simulink model "rev1BB"  (R2021a)
settings: Solver=FixedStepAuto  StartTime=0.0  StopTime=((((preLen+100+dataLenSymbols)*1+pad_first*3)*basePer))*2.5  RelTol=1e-3
values from neighbouring files (symbols this model uses):
  agcDesired = 0    [rev1BB_setup.m]
  agcStep = 2^-8    (= 0.00390625)    [rev1BB_setup.m]
  awgnSeed = abs(dBSnrRange(dBSnrInd)*1000+trial+10000000)    [plotBer.m]    (also in plotBerParSim.m; rev1BB_startup.m = 67)
  basePer = 1/baseFreq    (= 5e-08)    [rev1BB_setup.m]
  bitsPerSymbolHeader = log2(radixHeader)    [rev1BB_setup.m]
  bitsPerSymbolMax = log2(radixMax)    [rev1BB_setup.m]
  cefEarlyWarning = 256    [rev1BB_setup.m]
  cefLen = length(x_CEF)    [rev1BB_setup.m]
  cfoNcoWordLen = 16    [rev1BB_setup.m]
  channelFIR = zeros(1, round(maxSampleDelay)+1)    [rev1BB_simParams_setup.m]
  corr_peak_exclude_trigger = 1+corr_peak_trigger    (= 1.4)    [rev1BB_setup.m]
  corr_peak_trigger = 0.40    (= 0.4)    [rev1BB_setup.m]
  cr_i = 0.020    (= 0.02)    [rev1BB_setup.m]
  cr_i_preamp = 2^-9    (= 0.001953125)    [rev1BB_setup.m]
  cr_p = 0.015    [rev1BB_setup.m]
  dataLenSymbols = header_len_bytes*8/bitsPerSymbolHeader + frame_len_bytes*8/bitsPerSymbol    [rev1BB_setup.m]
  enableTRFreqCorrection = true    [rev1BB_setup.m]
  freeze_agc_in_CEF = true    [rev1BB_setup.m]
  freeze_agc_in_HeaderPayload = true    [rev1BB_setup.m]
  freeze_fineCFO_in_CEF = false    [rev1BB_setup.m]
  freeze_fineCFO_in_HeaderPayload = false    [rev1BB_setup.m]
  golay_type = golayType    (= 32)    [rev1BB_setup.m]
  golayType = 32    [rev1BB_setup.m]
  lmsEqDepth = 16    [rev1BB_setup.m]
  lmsStep_meta = (lmsStep_final - lmsStep_init)/cefLen    [rev1BB_setup.m]
  manChan = false    [rev1BB_simParams_setup.m]
  minSTFPeaks = 3    [rev1BB_setup.m]
  modBPS = [1, 2, 4]    [rev1BB_setup.m]
  modKeys = [0, 1, 2]    [rev1BB_setup.m]
  overSample = 3    [berCurve.m]    (also in rev1BB_setup.m = 4)
  qam16_demod_scale_factor = qam16_hdl_distance/qam16_power_normalized_distance    [rev1BB_setup.m]
  rcRxFilt = rcSqrtFilt    [rev1BB_setup.m]
  rcTxFilt = rcSqrtFilt    [rev1BB_setup.m]
  RxAGCCorrectionLoopPartition = 3    [rev1BB_setup.m]
  RxAGCPwrAvgPartition = 2    [rev1BB_setup.m]
  RxCoarseCFOPartition = 13    [rev1BB_setup.m]
  RxDemodPartition = 15    [rev1BB_setup.m]
  RxEQPartition = 14    [rev1BB_setup.m]
  RxFeedbackPipelining = 64*16    (= 1024)    [rev1BB_setup.m]
  RxFineCFOPartition = 15    [rev1BB_setup.m]
  RxFreezeControllerPartition = 17    [rev1BB_setup.m]
  RxFreezeFeedbackPipelining = RxFeedbackPipelining    (= 1024)    [rev1BB_setup.m]
  RxHeaderDemodPartition = 15    [rev1BB_setup.m]
  RxHeaderParsePartition = 15    [rev1BB_setup.m]
  RxPackerPartition = 16    [rev1BB_setup.m]
  RxPacketControllerPartition = 17    [rev1BB_setup.m]
  RxRRCPartition = 1    [rev1BB_setup.m]
  RxTimingRecoveryControlPartition = 8    [rev1BB_setup.m]
  RxTimingRecoveryDelayAccumPartition = 10    [rev1BB_setup.m]
  RxTimingRecoveryEarlyLatePartition = 10    [rev1BB_setup.m]
  RxTimingRecoveryFreqEstPartition = 10    [rev1BB_setup.m]
  RxTimingRecoveryGolayCorrelatorPartition = 6    [rev1BB_setup.m]
  RxTimingRecoveryGolayPeakDetectPartition = 7    [rev1BB_setup.m]
  RxTimingRecoverySymbolClockPartition = 9    [rev1BB_setup.m]
  RxTimingRecoveryVariableDelayPartition = 5    [rev1BB_setup.m]
  timing_cefEarlyWarningTollerance = 5    [rev1BB_setup.m]
  timing_correlator_pipeline = 1    [rev1BB_setup.m]
  timing_differentiator_grpDelay_roundUp = ceil((timing_differentiator_len)/2+timing_differentiator_pipeline)    [rev1BB_setup.m]
  timing_differentiator_pipeline = 1    [rev1BB_setup.m]
  timing_p = -0.215    [rev1BB_setup.m]
  timing_tolerance = 4    [rev1BB_setup.m]
  timingDifferentiatorFilt = timingDifferentiatorFiltObj.Coefficients    [rev1BB_setup.m]
  timingMaxSymbols = dataLenSymbols + length(x_CEF) + length(x_STF)/x_STFRepCount*2+100    [rev1BB_setup.m]
  timingRecoveryDoneSamplesEarly = floor(RxFeedbackPipelining/overSample) - delayToOutputFromDataFSM-1    [rev1BB_setup.m]
  timingRecoveryFreqCorrectionAvgLen = 32    [rev1BB_setup.m]
  timingRecoveryFreqCorrectionDiscardLastN = 2    [rev1BB_setup.m]
  trEarlyLateIGain = -0.000000050    (= -5e-08)    [rev1BB_setup.m]
  trEarlyLatePGain = -0.00225    [rev1BB_setup.m]
  trFarrowTaps = 4    [rev1BB_setup.m]
  trFeedbackPipelining = 64*8    (= 512)    [rev1BB_setup.m]
  trIntPhaseCounterInit = mod(timing_differentiator_grpDelay_roundUp, overSample)    [rev1BB_setup.m]
  trMatch = mod(-trLenToFSM, overSample)    [rev1BB_setup.m]
  trTappedDelayLen = trTappedDelayBase+trFarrowTaps    (= 44)    [rev1BB_setup.m]
  tx_rx_gain = 1    [rev1BB_simParams_setup.m]
  TxResampleModulatorPartition = 1    [rev1BB_setup.m]
  TxRRCFilterPartition = 2    [rev1BB_setup.m]
  txTimingOffset = 0    [plotBer.m]    (also in plotBerParSim.m; rev1BB_startup.m = 2e-05)
  txTimingPhase = channelizerUpDownSampling*overSample*4+1    [rev1BB_simParams_setup.m]
  x_CEF = xSpectrum_CEF_short    [rev1BB_setup.m]
  x_STFRepCount = nSpectrum_STFRepCount_short    (= 60)    [rev1BB_setup.m]
undefined symbols (not defined in the file or in its folder): doppler, magnitude
libraries: simulink x29, rev1CyclopsLib x20, commdigbbndpm3 x9, dspsigops x6, commdigbbndam3 x4, hdlsllib x2, commchan3 x2, commrflib2 x1
(part 2 of 3)

== system rev1BB/receiver/SymbolDomainOuter/VITIS_CLOCK_DOMAIN_SymbolDomain/Demod ==
  symbolIn : Inport
  modulationMode : Inport  Port=2
  BPSK Demodulator Baseband : commdigbbndpm3/BPSK Demodulator Baseband  DecType=Hard decision  VarSource=Dialog  Variance=1  Ph=0  outDtype=uint8  derotateFactorWordLen=16  derotateFactorDataTypeStr=Inherit: Same word length as input  derotateFactorLastDataTypeStr=Inherit: Same word length as input
  Gain : Gain  Gain=qam16_demod_scale_factor
  Multiport Switch : MultiPortSwitch  DataPortOrder=Zero-based contiguous  zeroidx=on
  QPSK Demodulator Baseband : commdigbbndpm3/QPSK Demodulator Baseband  OutType=Integer  DecType=Hard decision  VarSource=Dialog  Variance=1  Dec=Gray  Ph=pi/4  outDtype1=Inherit via internal rule  outDtype2=uint8  derotateFactorWordLen=16  derotateFactorDataTypeStr=Inherit: Same word length as input  derotateFactorLastDataTypeStr=Inherit: Same word length as input
  Rectangular QAM Demodulator Baseband : commdigbbndam3/Rectangular QAM Demodulator Baseband  M=16  OutType=Integer  DecType=Hard decision  VarSource=Dialog  Variance=1  Dec=Gray  Mapping=[0:15]  PowType=Min. distance between symbols  MinDist=qam16_hdl_distance  AvgPow=1  PeakPow=1  Ph=0  outDtype1=Inherit via internal rule  outDtype2=uint8  derotateFactorWordLen=16  derotateFactorDataTypeStr=Inherit: Same word length as input  derotateFactorLastDataTypeStr=Inherit: Same word length as input  denormFactorWordLen=16  denormFactorDataTypeStr=Inherit: Same word length as input  denormFactorLastDataTypeStr=Inherit: Same word length as input  prodOutWordLen=32  prodOutOverflowMode=Wrap  prodOutRoundingMode=Floor  prodOutOvFlMode=off  prodOutOvFlModeLastStrValue=off  sumWordLen=32
  Terminator2 : Terminator
  VITIS_PARTITION : Constant  Value=RxDemodPartition
  demodOut : Outport
  wires:
  symbolIn/1 -> Gain/1, QPSK Demodulator Baseband/1, BPSK Demodulator Baseband/1
  Gain/1 -> Rectangular QAM Demodulator Baseband/1
  Multiport Switch/1 -> demodOut/1
  BPSK Demodulator Baseband/1 -> Multiport Switch/2
  QPSK Demodulator Baseband/1 -> Multiport Switch/3
  Rectangular QAM Demodulator Baseband/1 -> Multiport Switch/4
  modulationMode/1 -> Multiport Switch/1
  VITIS_PARTITION/1 -> Terminator2/1

== system rev1BB/receiver/SymbolDomainOuter/VITIS_CLOCK_DOMAIN_SymbolDomain/DownsampleCorrelator ==
  In1 : Inport
  In2 : Inport  Port=2
  In3 : Inport  Port=3
  Downsample1 : DownSample  N=overSample  RateOptions=Allow multirate processing
  Downsample2 : DownSample  N=overSample  RateOptions=Allow multirate processing
  Downsample3 : DownSample  N=overSample  RateOptions=Allow multirate processing
  Terminator2 : Terminator
  VITIS_PARTITION : Constant  Value=RxTimingRecoverySymbolClockPartition
  Out1 : Outport
  Out2 : Outport  Port=2
  Out3 : Outport  Port=3
  wires:
  In2/1 -> Downsample2/1
  In1/1 -> Downsample1/1
  Downsample3/1 -> Out3/1
  Downsample2/1 -> Out2/1
  In3/1 -> Downsample3/1
  Downsample1/1 -> Out1/1
  VITIS_PARTITION/1 -> Terminator2/1

== system rev1BB/receiver/SymbolDomainOuter/VITIS_CLOCK_DOMAIN_SymbolDomain/DownsampleSymbol ==
  In1 : Inport
  Downsample : DownSample  N=overSample  RateOptions=Allow multirate processing
  Terminator2 : Terminator
  VITIS_PARTITION : Constant  Value=RxTimingRecoverySymbolClockPartition
  Out1 : Outport
  wires:
  In1/1 -> Downsample/1
  Downsample/1 -> Out1/1
  VITIS_PARTITION/1 -> Terminator2/1

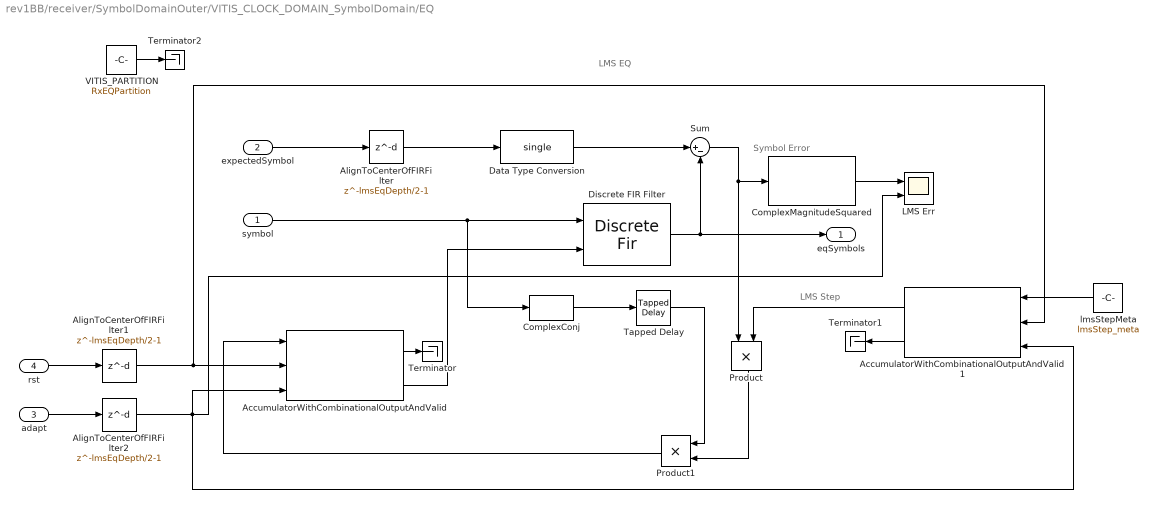
== system rev1BB/receiver/SymbolDomainOuter/VITIS_CLOCK_DOMAIN_SymbolDomain/EQ ==
  note: Symbol Error
  note: LMS EQ
  note: LMS Step
  symbol : Inport
  expectedSymbol : Inport  Port=2
  adapt : Inport  Port=3
  rst : Inport  Port=4
  AccumulatorWithCombinationalOutputAndValid : rev1CyclopsLib/AccumulatorWithCombinationalOutputAndValid  ResetVal=complex(cat(1,zeros(lmsEqDepth/2-1,1), [1], zeros(lmsEqDepth/2,1)))
  AccumulatorWithCombinationalOutputAndValid1 : rev1CyclopsLib/AccumulatorWithCombinationalOutputAndValid  ResetVal=lmsStep_init
  AlignToCenterOfFIRFilter : Delay  DelayLength=lmsEqDepth/2-1  UseCircularBuffer=on
  AlignToCenterOfFIRFilter1 : Delay  DelayLength=lmsEqDepth/2-1  UseCircularBuffer=on
  AlignToCenterOfFIRFilter2 : Delay  DelayLength=lmsEqDepth/2-1  UseCircularBuffer=on
  ComplexConj : rev1CyclopsLib/ComplexConj  SystemSampleTime=-1  VariantActivationTime=update diagram  Latency=0  AutoFrameSizeCalculation=off
  ComplexMagnitudeSquared : rev1CyclopsLib/ComplexMagnitudeSquared  SystemSampleTime=-1  VariantActivationTime=update diagram  Latency=0  AutoFrameSizeCalculation=off
  Data Type Conversion : DataTypeConversion  OutDataTypeStr=single
  Discrete FIR Filter : DiscreteFir  CoefSource=Input port
      settings: InputPortMap=u0,u1
  LMS Err : Scope  NumInputPorts=2
  Product : Product  OutDataTypeStr=Inherit: Same as first input
  Product1 : Product  OutDataTypeStr=Inherit: Same as first input
  Sum : Sum  Inputs=|+-  OutDataTypeStr=Inherit: Same as first input
  Tapped Delay : simulink/Discrete/Tapped Delay  vinit=0.0  samptime=-1  NumDelays=lmsEqDepth-1  DelayOrder=Newest  includeCurrent=on
  Terminator : Terminator
  Terminator1 : Terminator
  Terminator2 : Terminator
  VITIS_PARTITION : Constant  Value=RxEQPartition
  lmsStepMeta : Constant  Value=lmsStep_meta  OutDataTypeStr=single
  eqSymbols : Outport
  wires:
  Tapped Delay/1 -> Product1/1
  Discrete FIR Filter/1 -> eqSymbols/1, Sum/2
  ComplexConj/1 -> Tapped Delay/1
  AccumulatorWithCombinationalOutputAndValid/2 -> Discrete FIR Filter/2
  Product1/1 -> AccumulatorWithCombinationalOutputAndValid/1
  lmsStepMeta/1 -> AccumulatorWithCombinationalOutputAndValid1/1
  symbol/1 -> ComplexConj/1, Discrete FIR Filter/1
  Product/1 -> Product1/2
  AccumulatorWithCombinationalOutputAndValid/1 -> Terminator/1
  rst/1 -> AlignToCenterOfFIRFilter1/1
  expectedSymbol/1 -> AlignToCenterOfFIRFilter/1
  AccumulatorWithCombinationalOutputAndValid1/2 -> Terminator1/1
  AlignToCenterOfFIRFilter/1 -> Data Type Conversion/1
  AlignToCenterOfFIRFilter2/1 -> LMS Err/2, AccumulatorWithCombinationalOutputAndValid/3, AccumulatorWithCombinationalOutputAndValid1/3
  AlignToCenterOfFIRFilter1/1 -> AccumulatorWithCombinationalOutputAndValid1/2, AccumulatorWithCombinationalOutputAndValid/2
  adapt/1 -> AlignToCenterOfFIRFilter2/1
  VITIS_PARTITION/1 -> Terminator2/1
  Data Type Conversion/1 -> Sum/1
  Sum/1 -> ComplexMagnitudeSquared/1, Product/1
  AccumulatorWithCombinationalOutputAndValid1/1 -> Product/2
  ComplexMagnitudeSquared/1 -> LMS Err/1

== system rev1BB/receiver/SymbolDomainOuter/VITIS_CLOCK_DOMAIN_SymbolDomain/EnabledSubsystemInputPipelining ==
  Cb_within_peak_range_in : Inport
  Cb_in : Inport  Port=2
  Ca_within_peak_range_in : Inport  Port=3
  DelayCorrRelToSymbol : Delay  DelayLength=1
  DelayCorrRelToSymbol1 : Delay  DelayLength=1
  DelayCorrRelToSymbol2 : Delay  DelayLength=1
  Terminator2 : Terminator
  VITIS_PARTITION : Constant  Value=RxTimingRecoverySymbolClockPartition
  Cb_within_peak_range_out : Outport
  Cb_out : Outport  Port=2
  Ca_within_peak_range_out : Outport  Port=3
  wires:
  Cb_in/1 -> DelayCorrRelToSymbol1/1
  DelayCorrRelToSymbol1/1 -> Cb_out/1
  Cb_within_peak_range_in/1 -> DelayCorrRelToSymbol/1
  Ca_within_peak_range_in/1 -> DelayCorrRelToSymbol2/1
  DelayCorrRelToSymbol2/1 -> Ca_within_peak_range_out/1
  DelayCorrRelToSymbol/1 -> Cb_within_peak_range_out/1
  VITIS_PARTITION/1 -> Terminator2/1

== system rev1BB/receiver/SymbolDomainOuter/VITIS_CLOCK_DOMAIN_SymbolDomain/FineCFOCorrect ==
  symbolIn : Inport
  modulationMode : Inport  Port=2
  freezeCFO : Inport  Port=3
  cefDoneEarlyWarning : Inport  Port=4
  rst : Inport  Port=5
  AND : Logic  IconShape=distinctive  AllPortsSameDT=off  OutDataTypeStr=boolean
  Complex Exp : Subsystem
  EstPhase : Subsystem
  Fine CFO : Scope
  Loop Filter : Subsystem
  NOT : Logic  Operator=NOT  IconShape=distinctive  AllPortsSameDT=off  OutDataTypeStr=boolean
  PhaseCorrectionAccumulator : Subsystem
  Product : Product
  Terminator2 : Terminator
  VITIS_PARTITION : Constant  Value=RxFineCFOPartition
  checkIfInQuads2Or3 : Subsystem
  symbolCorrected : Outport
  wires:
  symbolIn/1 -> Product/1
  Product/1 -> symbolCorrected/1, EstPhase/1(symbol)
  modulationMode/1 -> EstPhase/2(modulationMode)
  EstPhase/1(phaseOffset) -> Loop Filter/1(phaseOffset)
  rst/1 -> PhaseCorrectionAccumulator/2(rst), Loop Filter/2(rst)
  freezeCFO/1 -> NOT/1
  NOT/1 -> Loop Filter/Enable
  Loop Filter/1(correction) -> PhaseCorrectionAccumulator/1(correction)
  PhaseCorrectionAccumulator/1(phaseCorrection) -> Fine CFO/1, checkIfInQuads2Or3/1(correction), Complex Exp/1(In1)
  Complex Exp/1(Out1) -> Product/2
  checkIfInQuads2Or3/1(inQuads23) -> AND/1
  cefDoneEarlyWarning/1 -> AND/2
  AND/1 -> PhaseCorrectionAccumulator/3(shift180)
  VITIS_PARTITION/1 -> Terminator2/1

== system rev1BB/receiver/SymbolDomainOuter/VITIS_CLOCK_DOMAIN_SymbolDomain/FreezeController ==
  inCEF : Inport
  inHeaderPayload : Inport  Port=2
  AND{,1..3} (4 alike) : Logic  IconShape=distinctive  AllPortsSameDT=off  OutDataTypeStr=boolean
  OR : Logic  Operator=OR  IconShape=distinctive  AllPortsSameDT=off  OutDataTypeStr=boolean
  OR1 : Logic  Operator=OR  IconShape=distinctive  AllPortsSameDT=off  OutDataTypeStr=boolean
  Terminator2 : Terminator
  VITIS_PARTITION : Constant  Value=RxFreezeControllerPartition
  freeze_agc_in_CEF : Constant  Value=freeze_agc_in_CEF  OutDataTypeStr=boolean
  freeze_agc_in_HeaderPayload : Constant  Value=freeze_agc_in_HeaderPayload  OutDataTypeStr=boolean
  freeze_fineCFO_in_CEF : Constant  Value=freeze_fineCFO_in_CEF  OutDataTypeStr=boolean
  freeze_fineCFO_in_HeaderPayload : Constant  Value=freeze_fineCFO_in_HeaderPayload  OutDataTypeStr=boolean
  freezeAGC : Outport
  freezeFineCFO : Outport  Port=2
  wires:
  freeze_agc_in_CEF/1 -> AND/1
  freeze_agc_in_HeaderPayload/1 -> AND1/1
  AND/1 -> OR/1
  AND1/1 -> OR/2
  OR/1 -> freezeAGC/1
  inHeaderPayload/1 -> AND3/2, AND1/2
  freeze_fineCFO_in_HeaderPayload/1 -> AND3/1
  inCEF/1 -> AND2/2, AND/2
  AND3/1 -> OR1/2
  freeze_fineCFO_in_CEF/1 -> AND2/1
  AND2/1 -> OR1/1
  VITIS_PARTITION/1 -> Terminator2/1
  OR1/1 -> freezeFineCFO/1

== system rev1BB/receiver/SymbolDomainOuter/VITIS_CLOCK_DOMAIN_SymbolDomain/FreezeControllerUpsample ==
  In1 : Inport
  Repeat1 : dspsigops/Repeat  N=overSample  RateOptions=Allow multirate processing  ic=0  mode=Unused parameter value
      settings: SourceProductName=DSP System Toolbox
  Terminator2 : Terminator
  VITIS_PARTITION : Constant  Value=RxFreezeControllerPartition
  Out1 : Outport
  wires:
  Repeat1/1 -> Out1/1
  In1/1 -> Repeat1/1
  VITIS_PARTITION/1 -> Terminator2/1

== system rev1BB/receiver/SymbolDomainOuter/VITIS_CLOCK_DOMAIN_SymbolDomain/HeaderDemod ==
  symbolIn : Inport
  BPSK Demodulator Baseband : commdigbbndpm3/BPSK Demodulator Baseband  DecType=Hard decision  VarSource=Dialog  Variance=1  Ph=0  outDtype=uint8  derotateFactorWordLen=16  derotateFactorDataTypeStr=Inherit: Same word length as input  derotateFactorLastDataTypeStr=Inherit: Same word length as input
  Terminator2 : Terminator
  VITIS_PARTITION : Constant  Value=RxHeaderDemodPartition
  demodOut : Outport
  wires:
  symbolIn/1 -> BPSK Demodulator Baseband/1
  BPSK Demodulator Baseband/1 -> demodOut/1
  VITIS_PARTITION/1 -> Terminator2/1

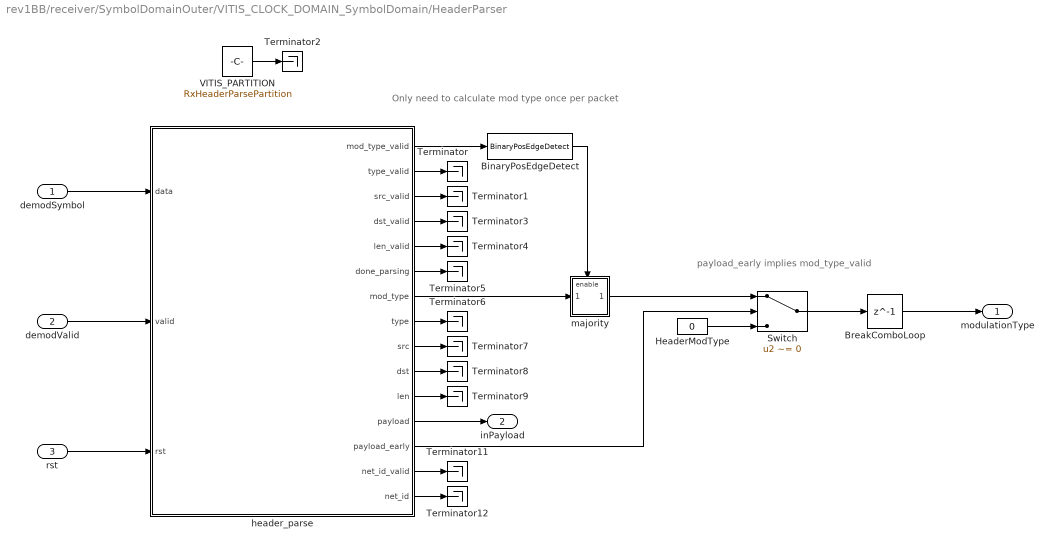
== system rev1BB/receiver/SymbolDomainOuter/VITIS_CLOCK_DOMAIN_SymbolDomain/HeaderParser ==
  note: Only need to calculate mod type once per packet
  note: payload_early implies mod_type_valid
  demodSymbol : Inport
  demodValid : Inport  Port=2
  rst : Inport  Port=3
  BinaryPosEdgeDetect : rev1CyclopsLib/BinaryPosEdgeDetect  SystemSampleTime=-1  VariantActivationTime=update diagram  Latency=0  AutoFrameSizeCalculation=off
  BreakComboLoop : Delay  DelayLength=1
  HeaderModType : Constant  Value=0  OutDataTypeStr=Inherit: Inherit via back propagation
  Switch : Switch  Criteria=u2 ~= 0
  Terminator{,1..9,11..12} (12 alike) : Terminator
  VITIS_PARTITION : Constant  Value=RxHeaderParsePartition
  header_parse : Stateflow chart  TreatAsAtomicUnit=on
  majority : Subsystem
  modulationType : Outport
  inPayload : Outport  Port=2
  wires:
  VITIS_PARTITION/1 -> Terminator2/1
  demodSymbol/1 -> header_parse/1(data)
  demodValid/1 -> header_parse/2(valid)
  rst/1 -> header_parse/3(rst)
  HeaderModType/1 -> Switch/3
  Switch/1 -> BreakComboLoop/1
  header_parse/7(mod_type) -> majority/1(In1)
  majority/1(Out1) -> Switch/1
  header_parse/1(mod_type_valid) -> BinaryPosEdgeDetect/1
  BinaryPosEdgeDetect/1 -> majority/Enable
  header_parse/13(payload_early) -> Switch/2
  header_parse/2(type_valid) -> Terminator/1
  header_parse/15(net_id) -> Terminator12/1
  header_parse/14(net_id_valid) -> Terminator11/1
  header_parse/12(payload) -> inPayload/1
  header_parse/11(len) -> Terminator9/1
  header_parse/10(dst) -> Terminator8/1
  header_parse/9(src) -> Terminator7/1
  header_parse/8(type) -> Terminator6/1
  header_parse/3(src_valid) -> Terminator1/1
  header_parse/4(dst_valid) -> Terminator3/1
  header_parse/5(len_valid) -> Terminator4/1
  header_parse/6(done_parsing) -> Terminator5/1
  BreakComboLoop/1 -> modulationType/1

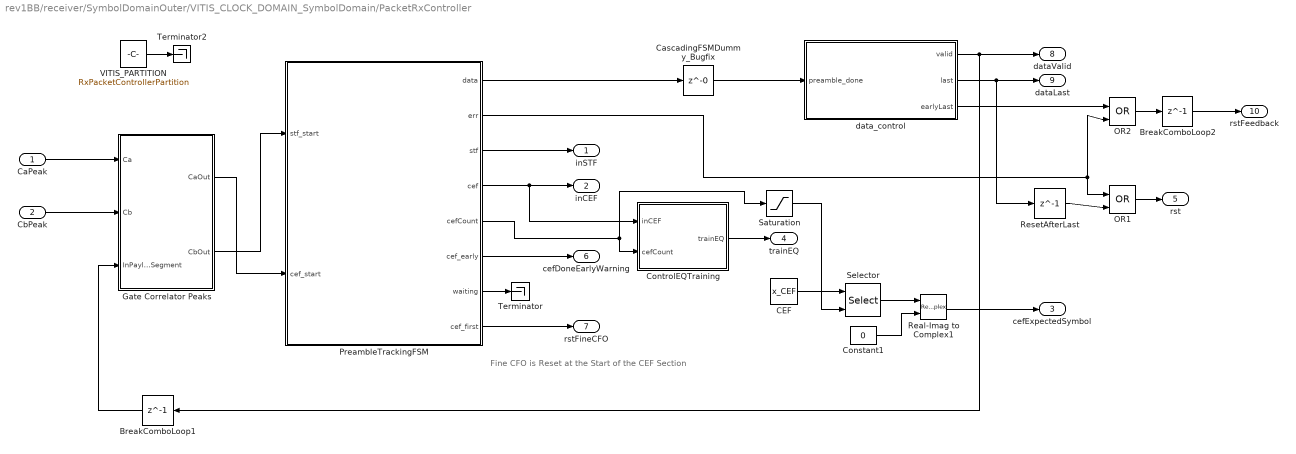
== system rev1BB/receiver/SymbolDomainOuter/VITIS_CLOCK_DOMAIN_SymbolDomain/PacketRxController ==
  note: Fine CFO is Reset at the Start of the CEF Section
  CaPeak : Inport
  CbPeak : Inport  Port=2
  BreakComboLoop1 : Delay  DelayLength=1
  BreakComboLoop2 : Delay  DelayLength=1
  CEF : Constant  Value=x_CEF  OutDataTypeStr=int16
  CascadingFSMDummy_Bugfix : Delay  DelayLength=0
  Constant1 : Constant  Value=0  OutDataTypeStr=Inherit: Inherit via back propagation
  ControlEQTraining : Subsystem
  Gate Correlator Peaks : Subsystem
  OR1 : Logic  Operator=OR  IconShape=distinctive  AllPortsSameDT=off  OutDataTypeStr=boolean
  OR2 : Logic  Operator=OR  IconShape=distinctive  AllPortsSameDT=off  OutDataTypeStr=boolean
  PreambleTrackingFSM : Stateflow chart  TreatAsAtomicUnit=on
  Real-Imag to Complex1 : RealImagToComplex
  ResetAfterLast : Delay  DelayLength=1
  Saturation : Saturate  UpperLimit=length(x_CEF)  LowerLimit=1
  Selector : Selector  InputPortWidth=length(x_CEF)  IndexOptions=Index vector (port)  Indices=[1 3]  OutputSizes=1
  Terminator : Terminator
  Terminator2 : Terminator
  VITIS_PARTITION : Constant  Value=RxPacketControllerPartition
  data_control : Stateflow chart  TreatAsAtomicUnit=on
  inSTF : Outport
  inCEF : Outport  Port=2
  cefExpectedSymbol : Outport  Port=3
  trainEQ : Outport  Port=4
  rst : Outport  Port=5
  cefDoneEarlyWarning : Outport  Port=6
  rstFineCFO : Outport  Port=7
  dataValid : Outport  Port=8
  dataLast : Outport  Port=9
  rstFeedback : Outport  Port=10
  wires:
  PreambleTrackingFSM/1(data) -> CascadingFSMDummy_Bugfix/1
  PreambleTrackingFSM/3(stf) -> inSTF/1
  PreambleTrackingFSM/4(cef) -> ControlEQTraining/1(inCEF), inCEF/1
  PreambleTrackingFSM/2(err) -> OR2/2, OR1/1
  data_control/1(valid) -> BreakComboLoop1/1, dataValid/1
  data_control/2(last) -> dataLast/1, ResetAfterLast/1
  data_control/3(earlyLast) -> OR2/1
  CaPeak/1 -> Gate Correlator Peaks/1(Ca)
  CbPeak/1 -> Gate Correlator Peaks/2(Cb)
  BreakComboLoop1/1 -> Gate Correlator Peaks/3(InPayloadSegment)
  Gate Correlator Peaks/1(CaOut) -> PreambleTrackingFSM/2(cef_start)
  Gate Correlator Peaks/2(CbOut) -> PreambleTrackingFSM/1(stf_start)
  ResetAfterLast/1 -> OR1/2
  OR1/1 -> rst/1
  ControlEQTraining/1(trainEQ) -> trainEQ/1
  PreambleTrackingFSM/5(cefCount) -> ControlEQTraining/2(cefCount), Saturation/1
  PreambleTrackingFSM/8(cef_first) -> rstFineCFO/1
  PreambleTrackingFSM/6(cef_early) -> cefDoneEarlyWarning/1
  PreambleTrackingFSM/7(waiting) -> Terminator/1
  OR2/1 -> BreakComboLoop2/1
  BreakComboLoop2/1 -> rstFeedback/1
  VITIS_PARTITION/1 -> Terminator2/1
  CascadingFSMDummy_Bugfix/1 -> data_control/1(preamble_done)
  CEF/1 -> Selector/1
  Selector/1 -> Real-Imag to Complex1/1
  Constant1/1 -> Real-Imag to Complex1/2
  Real-Imag to Complex1/1 -> cefExpectedSymbol/1
  Saturation/1 -> Selector/2

== system rev1BB/receiver/SymbolDomainOuter/VITIS_CLOCK_DOMAIN_SymbolDomain/PacketRxControllerUpsample ==
  In1 : Inport
  Repeat : dspsigops/Repeat  N=overSample  RateOptions=Allow multirate processing  ic=0  mode=Unused parameter value
      settings: SourceProductName=DSP System Toolbox
  Terminator2 : Terminator
  VITIS_PARTITION : Constant  Value=RxPacketControllerPartition
  Out1 : Outport
  wires:
  Repeat/1 -> Out1/1
  In1/1 -> Repeat/1
  VITIS_PARTITION/1 -> Terminator2/1

== system rev1BB/receiver/SymbolDomainOuter/VITIS_CLOCK_DOMAIN_SymbolDomain/dummyNode ==
  In1 : Inport
  DummyDelay : Delay  DelayLength=0
  Terminator2 : Terminator
  VITIS_PARTITION : Constant  Value=RxCoarseCFOPartition
  Out1 : Outport
  wires:
  DummyDelay/1 -> Out1/1
  In1/1 -> DummyDelay/1
  VITIS_PARTITION/1 -> Terminator2/1

== system rev1BB/receiver/TimingRecoveryAndCorrelator/EarlyLate/EarlyLateEst ==
  note: Early/Late Comparison
  pulseShapedCorr : Inport
  symbolClk : Inport  Port=2
  rst : Inport  Port=3
  Enable : EnablePort
  AccumulatorWithCombinationalOutputAndValid : rev1CyclopsLib/AccumulatorWithCombinationalOutputAndValid  ResetVal=0
  ComplexMagnitudeSquared : rev1CyclopsLib/ComplexMagnitudeSquared  SystemSampleTime=-1  VariantActivationTime=update diagram  Latency=0  AutoFrameSizeCalculation=off
  Delay : Delay
  I Gain1 : Gain  Gain=trEarlyLateIGain
  LateVsEarly : Subsystem
  OR : Logic  Operator=OR  IconShape=distinctive  AllPortsSameDT=off  OutDataTypeStr=boolean
  P Gain : Gain  Gain=trEarlyLatePGain
  Subtract : Sum  Inputs=+-  OutDataTypeStr=Inherit: Same as first input
  Sum : Sum  Inputs=|++  OutDataTypeStr=Inherit: Same as first input
  Terminator : Terminator
  earlyLateDelayCompensate1 : Delay  DelayLength=1
  earlyLateCorrection : Outport
  wires:
  ComplexMagnitudeSquared/1 -> Subtract/1, Delay/1
  Delay/1 -> Subtract/2
  Subtract/1 -> LateVsEarly/1(In1)
  LateVsEarly/1(Out1) -> AccumulatorWithCombinationalOutputAndValid/1, P Gain/1
  earlyLateDelayCompensate1/1 -> AccumulatorWithCombinationalOutputAndValid/3, OR/1
  rst/1 -> AccumulatorWithCombinationalOutputAndValid/2, LateVsEarly/2(rst), OR/2
  OR/1 -> LateVsEarly/Enable
  AccumulatorWithCombinationalOutputAndValid/1 -> I Gain1/1
  P Gain/1 -> Sum/1
  I Gain1/1 -> Sum/2
  Sum/1 -> earlyLateCorrection/1
  AccumulatorWithCombinationalOutputAndValid/2 -> Terminator/1
  symbolClk/1 -> earlyLateDelayCompensate1/1
  pulseShapedCorr/1 -> ComplexMagnitudeSquared/1

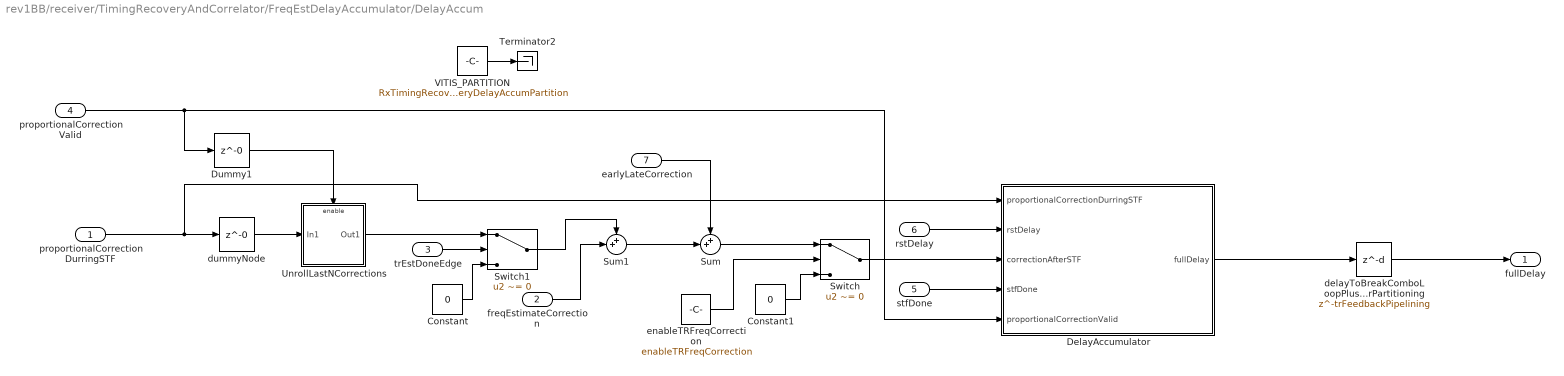
== system rev1BB/receiver/TimingRecoveryAndCorrelator/FreqEstDelayAccumulator/DelayAccum ==
  proportionalCorrectionDurringSTF : Inport
  freqEstimateCorrection : Inport  Port=2
  trEstDoneEdge : Inport  Port=3
  proportionalCorrectionValid : Inport  Port=4
  stfDone : Inport  Port=5
  rstDelay : Inport  Port=6
  earlyLateCorrection : Inport  Port=7
  Constant : Constant  Value=0  OutDataTypeStr=Inherit: Inherit via back propagation
  Constant1 : Constant  Value=0  OutDataTypeStr=Inherit: Inherit via back propagation
  DelayAccumulator : Subsystem
  Dummy1 : Delay  DelayLength=0
  Sum : Sum  Inputs=++|  OutDataTypeStr=Inherit: Same as first input
  Sum1 : Sum  Inputs=++|  OutDataTypeStr=Inherit: Same as first input
  Switch : Switch  Criteria=u2 ~= 0
  Switch1 : Switch  Criteria=u2 ~= 0
  Terminator2 : Terminator
  UnrollLastNCorrections : Subsystem
  VITIS_PARTITION : Constant  Value=RxTimingRecoveryDelayAccumPartition
  delayToBreakComboLoopPlusSlackForPartitioning : Delay  DelayLength=trFeedbackPipelining
  dummyNode : Delay  DelayLength=0
  enableTRFreqCorrection : Constant  Value=enableTRFreqCorrection
  fullDelay : Outport
  wires:
  stfDone/1 -> DelayAccumulator/4(stfDone)
  trEstDoneEdge/1 -> Switch1/2
  earlyLateCorrection/1 -> Sum/1
  Switch/1 -> DelayAccumulator/3(correctionAfterSTF)
  Switch1/1 -> Sum1/1
  Constant1/1 -> Switch/3
  Dummy1/1 -> UnrollLastNCorrections/Enable
  rstDelay/1 -> DelayAccumulator/2(rstDelay)
  UnrollLastNCorrections/1(Out1) -> Switch1/1
  Constant/1 -> Switch1/3
  enableTRFreqCorrection/1 -> Switch/2
  Sum/1 -> Switch/1
  freqEstimateCorrection/1 -> Sum1/2
  proportionalCorrectionValid/1 -> Dummy1/1, DelayAccumulator/5(proportionalCorrectionValid)
  proportionalCorrectionDurringSTF/1 -> dummyNode/1, DelayAccumulator/1(proportionalCorrectionDurringSTF)
  Sum1/1 -> Sum/2
  VITIS_PARTITION/1 -> Terminator2/1
  delayToBreakComboLoopPlusSlackForPartitioning/1 -> fullDelay/1
  DelayAccumulator/1(fullDelay) -> delayToBreakComboLoopPlusSlackForPartitioning/1
  dummyNode/1 -> UnrollLastNCorrections/1(In1)

== system rev1BB/receiver/TimingRecoveryAndCorrelator/FreqEstDelayAccumulator/EstimateTimingFreqOffset ==
  toAvg : Inport
  clearLastN : Inport  Port=2
  rst : Inport  Port=3
  Enable : EnablePort
  Constant : Constant  Value=zeros(1, numToClear)  OutDataTypeStr=Inherit: Inherit via back propagation
  Constant1 : Constant  Value=zeros(1, avgOver)  OutDataTypeStr=Inherit: Inherit via back propagation
  Constant2 : Constant  Value=(ones(1, avgOver)./(avgOver-timingRecoveryFreqCorrectionDiscardLastN)).*scaleBy  OutDataTypeStr=Inherit: Inherit via back propagation
  Delay : Delay  DelayLength=1  InitialCondition=zeros(avgOver, 1)
  Dot Product : DotProduct  InputSameDT=on
  Selector : Selector  InputPortWidth=avgOver  IndexOptions=Starting index (dialog)  Indices=1  OutputSizes=avgOver-1
  Selector1 : Selector  InputPortWidth=avgOver  IndexOptions=Starting index (dialog)  Indices=numToClear+1  OutputSizes=avgOver-numToClear
  Switch : Switch  Criteria=u2 ~= 0
  Switch1 : Switch  Criteria=u2 ~= 0
  Vector Concatenate : Concatenate
  Vector Concatenate1 : Concatenate
  avg : Outport
  wires:
  toAvg/1 -> Vector Concatenate/1
  Selector/1 -> Vector Concatenate/2
  Delay/1 -> Selector1/1, Selector/1
  Vector Concatenate1/1 -> Switch/1
  Switch/1 -> Switch1/3
  clearLastN/1 -> Switch/2
  rst/1 -> Switch1/2
  Vector Concatenate/1 -> Switch/3
  Constant1/1 -> Switch1/1
  Constant2/1 -> Dot Product/2
  Switch1/1 -> Dot Product/1, Delay/1
  Dot Product/1 -> avg/1
  Constant/1 -> Vector Concatenate1/1
  Selector1/1 -> Vector Concatenate1/2

== system rev1BB/receiver/TimingRecoveryAndCorrelator/GolayPeakDetect/GolayCorrelator ==
  In1 : Inport
  GolayCorrelator32 : rev1CyclopsLib/GolayCorrelator32  sampPerSym=overSample
  Terminator2 : Terminator
  VITIS_PARTITION : Constant  Value=RxTimingRecoveryGolayCorrelatorPartition
  Ca : Outport
  Cb : Outport  Port=2
  wires:
  GolayCorrelator32/2 -> Cb/1
  GolayCorrelator32/1 -> Ca/1
  In1/1 -> GolayCorrelator32/1
  VITIS_PARTITION/1 -> Terminator2/1

== system rev1BB/receiver/TimingRecoveryAndCorrelator/SymbolClockOuter/CheckIfSamplePointChanged ==
  lastGolayPeriod : Inport
  newPeriodAvail : Inport  Port=2
  AND : Logic  IconShape=distinctive  AllPortsSameDT=off  OutDataTypeStr=boolean
  Compare To Constant : simulink/Logic and Bit Operations/Compare To Constant  relop=~=  const=golay_type*overSample  OutDataTypeStr=boolean
  samplePointChanged : Outport
  wires:
  lastGolayPeriod/1 -> Compare To Constant/1
  Compare To Constant/1 -> AND/1
  newPeriodAvail/1 -> AND/2
  AND/1 -> samplePointChanged/1

== system rev1BB/receiver/TimingRecoveryAndCorrelator/SymbolClockOuter/SymbolClock ==
  rstClk : Inport
  Compare To Zero : simulink/Logic and Bit Operations/Compare To Zero  relop=<=  OutDataTypeStr=boolean
  Constant : Constant  Value=0  OutDataTypeStr=Inherit: Inherit via back propagation
  Constant1 : Constant  Value=overSample  OutDataTypeStr=int8
  Constant2 : Constant  OutDataTypeStr=Inherit: Inherit via back propagation
  Delay : Delay  DelayLength=1
  Subtract : Sum  Inputs=+-  OutDataTypeStr=Inherit: Same as first input
  Switch : Switch  Criteria=u2 ~= 0
  Switch1 : Switch  Criteria=u2 ~= 0
  symbolClk : Outport
  wires:
  Delay/1 -> Switch/3
  Constant/1 -> Switch/1
  rstClk/1 -> Switch/2
  Switch1/1 -> Subtract/1
  Switch/1 -> Switch1/3, Compare To Zero/1
  Compare To Zero/1 -> Switch1/2, symbolClk/1
  Constant1/1 -> Switch1/1
  Subtract/1 -> Delay/1
  Constant2/1 -> Subtract/2

== system rev1BB/receiver/TimingRecoveryAndCorrelator/TRControl/edgeDetect ==
  In1 : Inport
  AND : Logic  IconShape=distinctive  AllPortsSameDT=off  OutDataTypeStr=boolean
  Delay : Delay  DelayLength=1
  NOT : Logic  Operator=NOT  IconShape=distinctive  AllPortsSameDT=off  OutDataTypeStr=boolean
  rst : Outport
  wires:
  Delay/1 -> NOT/1
  AND/1 -> rst/1
  NOT/1 -> AND/2
  In1/1 -> Delay/1, AND/1

== system rev1BB/receiver/TimingRecoveryAndCorrelator/VarDelayWithSampleAlignment/VarDelay ==
  note: with a fracDelay of 0, the farrow structure still has a delay of 1 sample
      | (coeffients of the passed FIR filter is [0, 1, 0, 0] which is equivalent to z^-1)
      | With a passthrough value allowed in the tapped delay, we can effectivly
      | pass a 0 delay signal to the fractional delay (the current sample and 4 previous
      | ones).  The fractional delay filter effectivly adds 1 + the fractional delay.
      | Therefore, we can support delays in the range of (1, tappedDelayLen-4+1+2).
      | The extra +2 is from the maximum fractional delay
  note: The length of the tapped delay does not include the current sample,
      | the ouput vector is 1 longer than the tapped delay length.
      |
      | Allowed index for tapped delay are (0, lenTappedDelay+1-farrowTaps)
  samples : Inport
  delay : Inport  Port=2  OutDataTypeStr=single
  Constant : Constant  OutDataTypeStr=Inherit: Inherit via back propagation
  Data Type Conversion : DataTypeConversion  OutDataTypeStr=int32
  Pipeline : Delay  DelayLength=1
  Pipeline1 : Delay
  Pipeline2 : Delay  DelayLength=1
  Saturation : Saturate  UpperLimit=trTappedDelayLen+1-trFarrowTaps  LowerLimit=0  LinearizeAsGain=off
  Selector : Selector  IndexMode=Zero-based  InputPortWidth=trTappedDelayLen+1  IndexOptions=Starting index (port)  Indices=[1 3]  OutputSizes=trFarrowTaps
  Subtract : Sum  Inputs=+-  OutDataTypeStr=Inherit: Same as first input
  Subtract1 : Sum  Inputs=+-  OutDataTypeStr=Inherit: Same as first input
  Tapped Delay : simulink/Discrete/Tapped Delay  vinit=0.0  samptime=-1  NumDelays=trTappedDelayLen  DelayOrder=Newest  includeCurrent=on
  VarDelayScope : Scope  NumInputPorts=3
  frac_delay_farrow_N-2_M-3_extState : Subsystem  AncestorBlock=rev1CyclopsLib/frac_delay_farrow_N-2_M-3_extState
  out : Outport  VectorParamsAs1DForOutWhenUnconnected=off
  wires:
  Data Type Conversion/1 -> Subtract1/2, VarDelayScope/2, Pipeline/1
  Subtract1/1 -> VarDelayScope/3, Pipeline1/1
  Constant/1 -> Subtract/2
  Saturation/1 -> Data Type Conversion/1, Subtract1/1, VarDelayScope/1
  Subtract/1 -> Saturation/1
  delay/1 -> Subtract/1
  Selector/1 -> Pipeline2/1
  Tapped Delay/1 -> Selector/1
  samples/1 -> Tapped Delay/1
  frac_delay_farrow_N-2_M-3_extState/1(out) -> out/1
  Pipeline/1 -> Selector/2
  Pipeline1/1 -> frac_delay_farrow_N-2_M-3_extState/2(fracDelay)
  Pipeline2/1 -> frac_delay_farrow_N-2_M-3_extState/1(samples)

== system rev1BB/transmitter_outer/transmitter/VITIS_CLOCK_DOMAIN_modulate/modulator ==
  symbols : Inport
  modulationMode : Inport  Port=2
  BPSK Modulator Baseband : commdigbbndpm3/BPSK Modulator Baseband  Ph=0  outDtype=single  outWordLen=16  outUDDataType=sfix(16)  outFracLenMode=Best precision  outFracLen=15  outDataTypeStr=single  outLastDataTypeStr=single
  Bitwise AND : simulink/Logic and Bit Operations/Bitwise Operator  logicop=AND  UseBitMask=off  NumInputPorts=2  BitMask=bin2dec('11011001')  BitMaskRealWorld=Stored Integer
  Bitwise AND1 : simulink/Logic and Bit Operations/Bitwise Operator  logicop=AND  UseBitMask=off  NumInputPorts=2  BitMask=bin2dec('11011001')  BitMaskRealWorld=Stored Integer
  Bitwise AND2 : simulink/Logic and Bit Operations/Bitwise Operator  logicop=AND  UseBitMask=off  NumInputPorts=2  BitMask=bin2dec('11011001')  BitMaskRealWorld=Stored Integer
  Constant2 : Constant  Value=bin2dec('000001')  OutDataTypeStr=Inherit: Inherit via back propagation
  Constant3 : Constant  Value=bin2dec('000011')  OutDataTypeStr=Inherit: Inherit via back propagation
  Constant4 : Constant  Value=bin2dec('001111')  OutDataTypeStr=Inherit: Inherit via back propagation
  Multiport Switch : MultiPortSwitch  DataPortOrder=Zero-based contiguous  zeroidx=on
  QPSK Modulator Baseband : commdigbbndpm3/QPSK Modulator Baseband  InType=Integer  Enc=Gray  Ph=pi/4  outDtype=single  outWordLen=16  outUDDataType=sfix(16)  outFracLenMode=Best precision  outFracLen=15  outDataTypeStr=single  outLastDataTypeStr=single
  Rectangular QAM Modulator Baseband : commdigbbndam3/Rectangular QAM Modulator Baseband  M=16  InType=Integer  Enc=Gray  Mapping=[0:15]  PowType=Average Power  MinDist=2  AvgPow=1  PeakPow=1  Ph=0  outDtype=single  outWordLen=16  outUDDataType=sfix(16)  outFracLenMode=Best precision  outFracLen=15  outDataTypeStr=single  outLastDataTypeStr=single
  modulatedSymbols : Outport
  wires:
  Multiport Switch/1 -> modulatedSymbols/1
  modulationMode/1 -> Multiport Switch/1
  Constant2/1 -> Bitwise AND/2
  Bitwise AND1/1 -> QPSK Modulator Baseband/1
  symbols/1 -> Bitwise AND/1, Bitwise AND1/1, Bitwise AND2/1
  Constant3/1 -> Bitwise AND1/2
  Rectangular QAM Modulator Baseband/1 -> Multiport Switch/4
  Bitwise AND2/1 -> Rectangular QAM Modulator Baseband/1
  QPSK Modulator Baseband/1 -> Multiport Switch/3
  Constant4/1 -> Bitwise AND2/2
  Bitwise AND/1 -> BPSK Modulator Baseband/1
  BPSK Modulator Baseband/1 -> Multiport Switch/2

== system rev1BB/receiver/SymbolDomainOuter/VITIS_CLOCK_DOMAIN_SymbolDomain/CoarseCFOCorrect/ApplyCorrection ==
  phaseIncrement : Inport
  symbolIn : Inport  Port=2
  Data Type Conversion : DataTypeConversion  OutDataTypeStr=int32
  NCO : dspsigops/NCO  AccIncSrc=Input port  AccInc=100  PhaseOffsetSrc=Specify via dialog  PhaseOffset=0  AccumWL=cfoNcoWordLen  HasDither=off  DitherWL=4  PNgeneratorLength=19  HasPhaseQuantizer=on  TableDepth=cfoNcoQuantizedAccumBits  HasOutputPhaseError=off  Formula=Complex exponential  DataType=single  OutputWL=16  OutputFL=14  CompMethod=Table lookup (no interpolation)  SampleTime=1  SamplesPerFrame=1  OutputFrames=off
      settings: SourceProductBaseCode=DS
  Product : Product
  symbolOut : Outport
  wires:
  Data Type Conversion/1 -> NCO/1
  phaseIncrement/1 -> Data Type Conversion/1
  NCO/1 -> Product/1
  symbolIn/1 -> Product/2
  Product/1 -> symbolOut/1

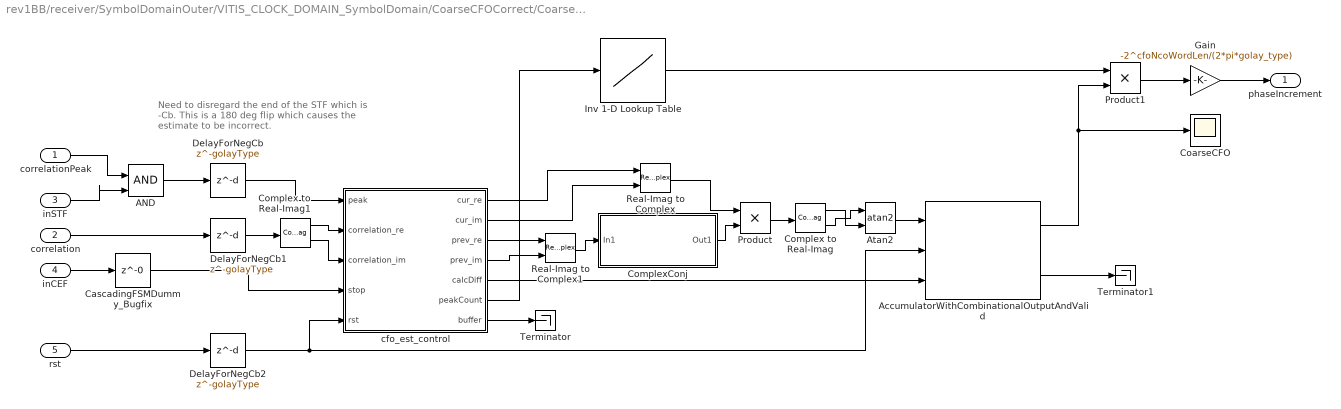
== system rev1BB/receiver/SymbolDomainOuter/VITIS_CLOCK_DOMAIN_SymbolDomain/CoarseCFOCorrect/CoarseCFOEstimate ==
  note: Need to disregard the end of
      | the STF which is -Cb.  This is a 180 deg flip
      | which causes the estimate to be incorrect.
  correlationPeak : Inport
  correlation : Inport  Port=2
  inSTF : Inport  Port=3
  inCEF : Inport  Port=4
  rst : Inport  Port=5
  AND : Logic  IconShape=distinctive  AllPortsSameDT=off  OutDataTypeStr=boolean
  AccumulatorWithCombinationalOutputAndValid : rev1CyclopsLib/AccumulatorWithCombinationalOutputAndValid  ResetVal=0
  Atan2 : Trigonometry  Operator=atan2
  CascadingFSMDummy_Bugfix : Delay  DelayLength=0
  CoarseCFO : Scope
  Complex to Real-Imag : ComplexToRealImag
  Complex to Real-Imag1 : ComplexToRealImag
  ComplexConj : Subsystem
  DelayForNegCb : Delay  DelayLength=golayType
  DelayForNegCb1 : Delay  DelayLength=golayType
  DelayForNegCb2 : Delay  DelayLength=golayType
  Gain : Gain  Gain=-2^cfoNcoWordLen/(2*pi*golay_type)
  Inv 1-D Lookup Table : Lookup_n-D  NumberOfTableDimensions=1  BreakpointsForDimension1=[0:(x_STFRepCount+1)]  IndexSearchMethod=Evenly spaced points  Table=cat(2, [1], 1./[1:(x_STFRepCount+1)] )  InterpMethod=Flat  DiagnosticForOutOfRangeInput=Error  InternalRulePriority=Speed  OutDataTypeStr=single  RndMeth=Simplest  InputSameDT=on
  Product : Product  OutDataTypeStr=Inherit: Same as first input
  Product1 : Product  OutDataTypeStr=Inherit: Same as first input
  Real-Imag to Complex : RealImagToComplex
  Real-Imag to Complex1 : RealImagToComplex
  Terminator : Terminator
  Terminator1 : Terminator
  cfo_est_control : Stateflow chart  TreatAsAtomicUnit=on
  phaseIncrement : Outport
  wires:
  inCEF/1 -> CascadingFSMDummy_Bugfix/1
  rst/1 -> DelayForNegCb2/1
  ComplexConj/1(Out1) -> Product/2
  Product/1 -> Complex to Real-Imag/1
  Complex to Real-Imag/2 -> Atan2/1
  Complex to Real-Imag/1 -> Atan2/2
  cfo_est_control/6(peakCount) -> Inv 1-D Lookup Table/1
  cfo_est_control/5(calcDiff) -> AccumulatorWithCombinationalOutputAndValid/3
  cfo_est_control/7(buffer) -> Terminator/1
  Inv 1-D Lookup Table/1 -> Product1/1
  AccumulatorWithCombinationalOutputAndValid/1 -> CoarseCFO/1, Product1/2
  correlation/1 -> DelayForNegCb1/1
  inSTF/1 -> AND/2
  correlationPeak/1 -> AND/1
  AND/1 -> DelayForNegCb/1
  Product1/1 -> Gain/1
  Gain/1 -> phaseIncrement/1
  AccumulatorWithCombinationalOutputAndValid/2 -> Terminator1/1
  Atan2/1 -> AccumulatorWithCombinationalOutputAndValid/1
  DelayForNegCb1/1 -> Complex to Real-Imag1/1
  DelayForNegCb2/1 -> cfo_est_control/5(rst), AccumulatorWithCombinationalOutputAndValid/2
  cfo_est_control/1(cur_re) -> Real-Imag to Complex/1
  cfo_est_control/2(cur_im) -> Real-Imag to Complex/2
  Real-Imag to Complex/1 -> Product/1
  cfo_est_control/3(prev_re) -> Real-Imag to Complex1/1
  cfo_est_control/4(prev_im) -> Real-Imag to Complex1/2
  Real-Imag to Complex1/1 -> ComplexConj/1(In1)
  DelayForNegCb/1 -> cfo_est_control/1(peak)
  Complex to Real-Imag1/1 -> cfo_est_control/2(correlation_re)
  Complex to Real-Imag1/2 -> cfo_est_control/3(correlation_im)
  CascadingFSMDummy_Bugfix/1 -> cfo_est_control/4(stop)

== system rev1BB/receiver/SymbolDomainOuter/VITIS_CLOCK_DOMAIN_SymbolDomain/FineCFOCorrect/Complex Exp ==
  In1 : Inport
  Cos : Trigonometry  Operator=cos
  Real-Imag to Complex : RealImagToComplex
  Sin : Trigonometry
  Out1 : Outport
  wires:
  Sin/1 -> Real-Imag to Complex/2
  Real-Imag to Complex/1 -> Out1/1
  Cos/1 -> Real-Imag to Complex/1
  In1/1 -> Sin/1, Cos/1

== system rev1BB/receiver/SymbolDomainOuter/VITIS_CLOCK_DOMAIN_SymbolDomain/FineCFOCorrect/EstPhase ==
  symbol : Inport
  modulationMode : Inport  Port=2
  Atan2 : Trigonometry  Operator=atan2
  Complex to Real-Imag : ComplexToRealImag
  ComplexConj : rev1CyclopsLib/ComplexConj  SystemSampleTime=-1  VariantActivationTime=update diagram  Latency=0  AutoFrameSizeCalculation=off
  Product : Product  OutDataTypeStr=Inherit: Same as first input
  findNearestConstPt : Subsystem
  phaseOffset : Outport
  wires:
  symbol/1 -> ComplexConj/1, findNearestConstPt/1(symbol)
  modulationMode/1 -> findNearestConstPt/2(modulationMode)
  findNearestConstPt/1(nearestPt) -> Product/1
  ComplexConj/1 -> Product/2
  Product/1 -> Complex to Real-Imag/1
  Atan2/1 -> phaseOffset/1
  Complex to Real-Imag/2 -> Atan2/1
  Complex to Real-Imag/1 -> Atan2/2

== system rev1BB/receiver/SymbolDomainOuter/VITIS_CLOCK_DOMAIN_SymbolDomain/FineCFOCorrect/Loop Filter ==
  phaseOffset : Inport  PortDimensions=1
  rst : Inport  Port=2
  Enable : EnablePort
  AccumulatorWithDecaySaturationCombinationalOutput : rev1CyclopsLib/AccumulatorWithDecaySaturationCombinationalOutput  ResetVal=0  Decay=cr_integrator1_decay  SatUp=cr_int1_sat_up  SatDown=cr_int1_sat_low
  RollingAverage : rev1CyclopsLib/RollingAverage  averagingSamples=cr_smooth_samples
  Sum : Sum  Inputs=|++
  Terminator : Terminator
  cr_i : Gain  Gain=cr_i  OutDataTypeStr=Inherit: Same as input
  cr_i_preamp : Gain  Gain=cr_i_preamp  OutDataTypeStr=Inherit: Same as input
  cr_p : Gain  Gain=cr_p  OutDataTypeStr=Inherit: Same as input
  correction : Outport
  wires:
  phaseOffset/1 -> RollingAverage/1
  RollingAverage/1 -> cr_i_preamp/1, cr_p/1
  cr_i_preamp/1 -> AccumulatorWithDecaySaturationCombinationalOutput/1
  rst/1 -> AccumulatorWithDecaySaturationCombinationalOutput/2
  AccumulatorWithDecaySaturationCombinationalOutput/1 -> cr_i/1
  AccumulatorWithDecaySaturationCombinationalOutput/2 -> Terminator/1
  cr_p/1 -> Sum/1
  cr_i/1 -> Sum/2
  Sum/1 -> correction/1

== system rev1BB/receiver/SymbolDomainOuter/VITIS_CLOCK_DOMAIN_SymbolDomain/FineCFOCorrect/PhaseCorrectionAccumulator ==
  note: Using the sequential output to break the correction
      | Combo Loop
  correction : Inport
  rst : Inport  Port=2
  shift180 : Inport  Port=3
  Constant : Constant  Value=0  OutDataTypeStr=Inherit: Inherit via back propagation
  Delay : Delay  DelayLength=1
  PreventPotentialOverflow : Saturate  UpperLimit=pi  LowerLimit=-pi
  PseudoFMod2Pi : Subsystem
  Shift180 : Subsystem
  Sum : Sum  Inputs=|++
  Switch : Switch  Criteria=u2 ~= 0
  phaseCorrection : Outport
  wires:
  correction/1 -> PreventPotentialOverflow/1
  shift180/1 -> Shift180/2(shift180)
  PreventPotentialOverflow/1 -> Shift180/1(correction)
  rst/1 -> Switch/2
  Switch/1 -> Delay/1
  Delay/1 -> Sum/2, phaseCorrection/1
  Constant/1 -> Switch/1
  Shift180/1(correctionOut) -> Sum/1
  PseudoFMod2Pi/1(Out1) -> Switch/3
  Sum/1 -> PseudoFMod2Pi/1(In1)

== system rev1BB/receiver/SymbolDomainOuter/VITIS_CLOCK_DOMAIN_SymbolDomain/FineCFOCorrect/checkIfInQuads2Or3 ==
  correction : Inport
  Compare To Constant : simulink/Logic and Bit Operations/Compare To Constant  relop=>  const=pi/2  OutDataTypeStr=boolean
  Compare To Constant1 : simulink/Logic and Bit Operations/Compare To Constant  relop=<  const=-pi/2  OutDataTypeStr=boolean
  OR : Logic  Operator=OR  IconShape=distinctive  AllPortsSameDT=off  OutDataTypeStr=boolean
  inQuads23 : Outport
  wires:
  Compare To Constant/1 -> OR/1
  OR/1 -> inQuads23/1
  correction/1 -> Compare To Constant/1, Compare To Constant1/1
  Compare To Constant1/1 -> OR/2

== system rev1BB/receiver/SymbolDomainOuter/VITIS_CLOCK_DOMAIN_SymbolDomain/HeaderParser/majority ==
  In1 : Inport
  Enable : EnablePort
  Bit Shift1 : hdlsllib/Logic and Bit Operations/Bit Shift  mode=Shift Right Logical  N=2
  Bit Shift2 : hdlsllib/Logic and Bit Operations/Bit Shift  mode=Shift Right Logical  N=4
  Bitwise AND : simulink/Logic and Bit Operations/Bitwise Operator  logicop=AND  UseBitMask=on  BitMask=bin2dec('00000011')  BitMaskRealWorld=Stored Integer
  Bitwise AND1 : simulink/Logic and Bit Operations/Bitwise Operator  logicop=AND  UseBitMask=on  BitMask=bin2dec('00000011')  BitMaskRealWorld=Stored Integer
  Bitwise AND2 : simulink/Logic and Bit Operations/Bitwise Operator  logicop=AND  UseBitMask=on  BitMask=bin2dec('00000011')  BitMaskRealWorld=Stored Integer
  Bitwise AND3 : simulink/Logic and Bit Operations/Bitwise Operator  logicop=AND  UseBitMask=off  NumInputPorts=2  BitMask=bin2dec('11011001')  BitMaskRealWorld=Stored Integer
  Bitwise AND4 : simulink/Logic and Bit Operations/Bitwise Operator  logicop=AND  UseBitMask=off  NumInputPorts=2  BitMask=bin2dec('11011001')  BitMaskRealWorld=Stored Integer
  Bitwise AND5 : simulink/Logic and Bit Operations/Bitwise Operator  logicop=AND  UseBitMask=off  NumInputPorts=2  BitMask=bin2dec('11011001')  BitMaskRealWorld=Stored Integer
  Bitwise OR : simulink/Logic and Bit Operations/Bitwise Operator  logicop=OR  UseBitMask=off  NumInputPorts=3  BitMask=bin2dec('11011001')  BitMaskRealWorld=Stored Integer
  Out1 : Outport
  wires:
  Bitwise OR/1 -> Out1/1
  Bitwise AND5/1 -> Bitwise OR/3
  Bit Shift1/1 -> Bitwise AND1/1
  Bit Shift2/1 -> Bitwise AND2/1
  Bitwise AND3/1 -> Bitwise OR/1
  Bitwise AND/1 -> Bitwise AND5/1, Bitwise AND3/1
  Bitwise AND1/1 -> Bitwise AND4/1, Bitwise AND3/2
  Bitwise AND4/1 -> Bitwise OR/2
  In1/1 -> Bit Shift2/1, Bit Shift1/1, Bitwise AND/1
  Bitwise AND2/1 -> Bitwise AND5/2, Bitwise AND4/2

== system rev1BB/receiver/SymbolDomainOuter/VITIS_CLOCK_DOMAIN_SymbolDomain/PacketRxController/ControlEQTraining ==
  note: Start adapting when in CEF. Stop adapting early to allow Fine CFO Correction to settle
  inCEF : Inport
  cefCount : Inport  Port=2
  AND : Logic  IconShape=distinctive  AllPortsSameDT=off  OutDataTypeStr=boolean
  Compare To Constant1 : simulink/Logic and Bit Operations/Compare To Constant  relop=<  const=cefLen-cefEarlyWarning  OutDataTypeStr=boolean
  trainEQ : Outport
  wires:
  cefCount/1 -> Compare To Constant1/1
  AND/1 -> trainEQ/1
  Compare To Constant1/1 -> AND/2
  inCEF/1 -> AND/1

== system rev1BB/receiver/SymbolDomainOuter/VITIS_CLOCK_DOMAIN_SymbolDomain/PacketRxController/Gate Correlator Peaks ==
  note: Pass if AGC settles or in preamble
      | Do not pass if in payload
  Ca : Inport
  Cb : Inport  Port=2
  InPayloadSegment : Inport  Port=3
  AND2 : Logic  IconShape=distinctive  AllPortsSameDT=off  OutDataTypeStr=boolean
  AND3 : Logic  IconShape=distinctive  AllPortsSameDT=off  OutDataTypeStr=boolean
  NOT : Logic  Operator=NOT  IconShape=distinctive  AllPortsSameDT=off  OutDataTypeStr=boolean
  CaOut : Outport
  CbOut : Outport  Port=2
  wires:
  InPayloadSegment/1 -> NOT/1
  Ca/1 -> AND2/1
  AND2/1 -> CaOut/1
  AND3/1 -> CbOut/1
  Cb/1 -> AND3/1
  NOT/1 -> AND3/2, AND2/2

== system rev1BB/receiver/TimingRecoveryAndCorrelator/EarlyLate/EarlyLateEst/LateVsEarly ==
  In1 : Inport
  rst : Inport  Port=2
  Enable : EnablePort
  RollingAverageWithReset : rev1CyclopsLib/RollingAverageWithReset  averagingSamples=trEarlyLateAvgNumSamp
  Out1 : Outport
  wires:
  In1/1 -> RollingAverageWithReset/1
  RollingAverageWithReset/1 -> Out1/1
  rst/1 -> RollingAverageWithReset/2

== system rev1BB/receiver/TimingRecoveryAndCorrelator/FreqEstDelayAccumulator/DelayAccum/DelayAccumulator ==
  proportionalCorrectionDurringSTF : Inport
  rstDelay : Inport  Port=2
  correctionAfterSTF : Inport  Port=3
  stfDone : Inport  Port=4
  proportionalCorrectionValid : Inport  Port=5
  AccumulatorWithCombinationalOutput : rev1CyclopsLib/AccumulatorWithCombinationalOutput  ResetVal=trInitialDelay
  Constant1 : Constant  Value=0  OutDataTypeStr=Inherit: Inherit via back propagation
  Switch1 : Switch  Criteria=u2 ~= 0
  Switch2 : Switch  Criteria=u2 ~= 0
  Terminator : Terminator
  fullDelay : Outport
  wires:
  proportionalCorrectionDurringSTF/1 -> Switch2/1
  Switch2/1 -> Switch1/3
  proportionalCorrectionValid/1 -> Switch2/2
  stfDone/1 -> Switch1/2
  correctionAfterSTF/1 -> Switch1/1
  rstDelay/1 -> AccumulatorWithCombinationalOutput/2
  Constant1/1 -> Switch2/3
  Switch1/1 -> AccumulatorWithCombinationalOutput/1
  AccumulatorWithCombinationalOutput/1 -> fullDelay/1
  AccumulatorWithCombinationalOutput/2 -> Terminator/1

== system rev1BB/receiver/TimingRecoveryAndCorrelator/FreqEstDelayAccumulator/DelayAccum/UnrollLastNCorrections ==
  In1 : Inport
  Enable : EnablePort
  Discrete FIR Filter : DiscreteFir  Coefficients=-1.*ones(1, timingRecoveryFreqCorrectionDiscardLastN)
  Out1 : Outport
  wires:
  Discrete FIR Filter/1 -> Out1/1
  In1/1 -> Discrete FIR Filter/1
